simulink model "reconfig"  (R2022a)
settings: Solver=VariableStepAuto  StartTime=0.0  StopTime=tsim  RelTol=1e-3
InitFcn:
  | main
values from neighbouring files (symbols this model uses):
  drone_params = get_parameters(3)    [main.m]
  dt = 0.005    [main.m]
  g = 9.81    [main.m]
  gust_duration = 5    [main.m]
  gust_force = [0;0;0]    [main.m]
  gust_start = 8    [main.m]
  omega0 = [[0,0,0]',[0,0,0]',[0,0,0]']    [main.m]
  p0 = [[0,0,2]',[0,0,2]',[0,0,2]']    [main.m]
  q0 = [[1,0,0,0]',[1,0,0,0]',[1,0,0,0]']    [main.m]
  v0 = [[0,0,0]',[0,0,0]',[0,0,0]']    [main.m]
undefined symbols (not defined in the file or in its folder): dThtdPhidPsi2pqr, pqr2dThtdPhidPsi
libraries: vrlib x1
settings Model: Creator=gbattaglia2021  LastModifiedBy=Giacomo Battaglia
settings DebuggingCC: UnconnectedInputMsg=warning  UnconnectedOutputMsg=warning  UnconnectedLineMsg=warning
settings RTWCC: DLArmComputeVersion=19.05

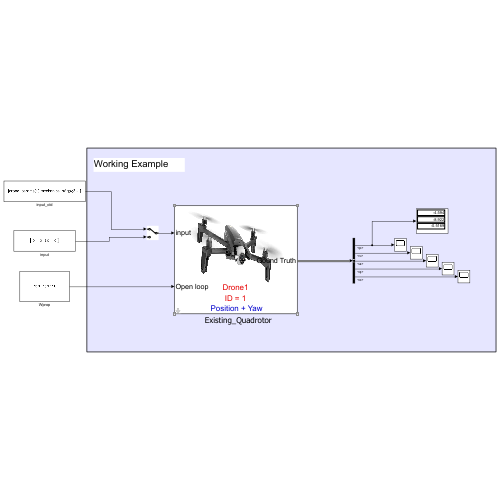
[thumbnail: Simulink's stored preview of the top-level diagram]
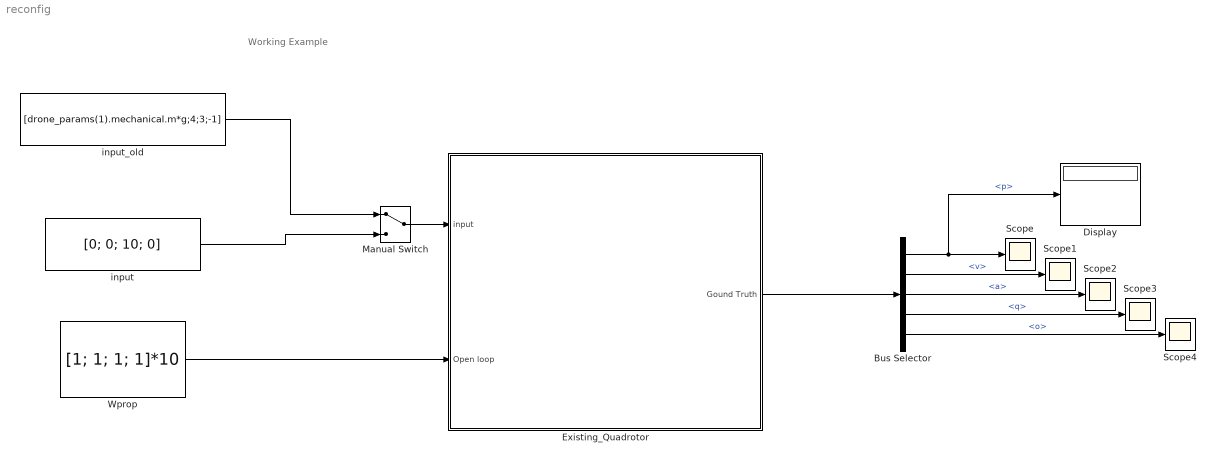
== system reconfig ==
  note: Working Example
  "  Existing_Quadrotor" : Subsystem  mask{control_type_param=1: Position + Yaw, DroneID=1, DroneName=Drone1, idx_offset=0}
      mask prompts: control_type_param "Controller type"; DroneName "Drone Name"; idx_offset "Index Offset"
      mask TypeOptions control_type_param: 1: Position + Yaw | 2: Body Velocity + Yawrate | 3: Body Acceleration + Yawrate | 4: Thrust + Attitude | 5: Thrust + Body Rate | 6: Body Wrench
      mask TypeOptions DroneID: 1 | 2 | 3 | 4 | 5 | 6 | 7 | 8 | 9
      mask Callback DroneID:
      | ID = get_param(gcb,'DroneID');
      | offset = get_param(gcb,'idx_offset');
      | if ischar(ID)
      |   ID = str2num(ID);
      | end
      | if ischar(offset)
      |   offset = str2num(offset);
      | end
      | nameID = ID + offset;
      | set_param(gcb,'DroneName',["Drone"+num2str(nameID)]);
      mask Callback DroneName: set_param([gcb,'/To Workspace'],'VariableName',[get_param(gcb,'DroneName')]);
      mask Callback idx_offset:
      | ID = get_param(gcb,'DroneID');
      | offset = get_param(gcb,'idx_offset');
      | if ischar(ID)
      |   ID = str2num(ID);
      | end
      | if ischar(offset)
      |   offset = str2num(offset);
      | end
      | nameID = ID + offset;
      | set_param(gcb,'DroneName',["Drone"+num2str(nameID)]);
      mask DialogControl Control4 Prompt: click to choose controller
      mask Display:
      | image('format/drone_image.png'); % Use "Edit Image" on toolstrip to change.
      | Name = get_param(gcb,'DroneName');
      | ID = get_param(gcb,'DroneID');
      | C_mode = get_param(gcb,'control_type_param');
      | C_mode(1:2) = [];
      | color('red')
      | ID = "ID = "+ID;
      | color('red')
      | text(0.5, 0.25, Name, 'horizontalAlignment', 'center')
      | color('red')
      | text(0.5, 0.15, ID, 'horizontalAlignment', 'center')
      | color('blue');
      | text(0.5, 0.05, C_mode, 'horizontalAlignment', 'center')
  Bus Selector : BusSelector  OutputSignals=p,v,a,q,o
  Display : Display
  Manual Switch : ManualSwitch
  Scope{,1..4} (5 alike) : Scope
  Wprop : Constant  Value=[1; 1; 1; 1]*10
  input : Constant  Value=[0; 0; 10; 0]
  input_old : Constant  Value=[drone_params(1).mechanical.m*g;4;3;-1]
  wires:
  Bus Selector/1 -> Display/1, Scope/1  "<p>"
  Bus Selector/4 -> Scope3/1  "<q>"
  Bus Selector/5 -> Scope4/1  "<o>"
  Bus Selector/2 -> Scope1/1  "<v>"
  "  Existing_Quadrotor"/1(Gound Truth) -> Bus Selector/1
  Bus Selector/3 -> Scope2/1  "<a>"
  Wprop/1 -> "  Existing_Quadrotor"/2(Open loop)
  Manual Switch/1 -> "  Existing_Quadrotor"/1(input)
  input_old/1 -> Manual Switch/1
  input/1 -> Manual Switch/2

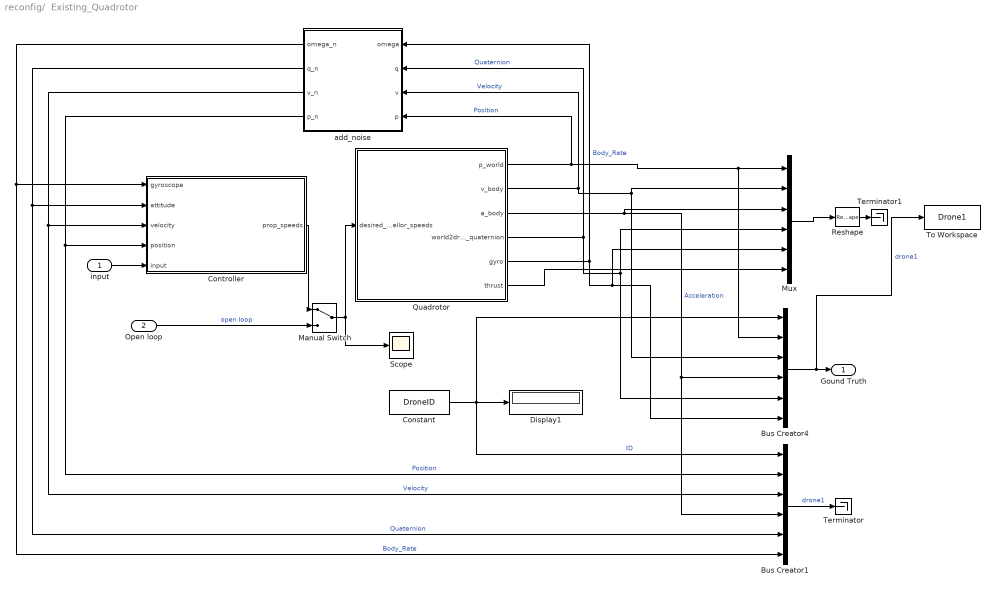
== system reconfig/  Existing_Quadrotor ==
  input : Inport
  Open loop : Inport  Port=2
  Bus Creator1 : BusCreator  Inputs=6  OutDataTypeStr=Bus: DroneStateBus
      settings: InheritFromInputs=off
  Bus Creator4 : BusCreator  Inputs=6  OutDataTypeStr=Bus: DroneStateBus
      settings: InheritFromInputs=off
  Constant : Constant  Value=DroneID
  Controller : Subsystem
  Display1 : Display
  Manual Switch : ManualSwitch
  Mux : Mux  Inputs=6
  Quadrotor : Subsystem
      mask Display: image('droneHardware.jpeg'); % Use "Edit Image" on toolstrip to change.
  Reshape : Reshape
  Scope : Scope
  Terminator : Terminator
  Terminator1 : Terminator
  To Workspace : ToWorkspace  VariableName=Drone1  SaveFormat=Timeseries  SampleTime=-1
  add_noise : MATLAB Function  TreatAsAtomicUnit=on
  Gound Truth : Outport
  wires:
  Quadrotor/5(gyro) -> add_noise/1(omega), Bus Creator4/6, Mux/5  "Body_Rate"
  Quadrotor/1(p_world) -> add_noise/4(p), Bus Creator4/2, Mux/1  "Position"
  Quadrotor/4(world2drone_quaternion) -> add_noise/2(q), Bus Creator4/5, Mux/4  "Quaternion"
  Mux/1 -> Reshape/1
  Quadrotor/2(v_body) -> add_noise/3(v), Bus Creator4/3, Mux/2  "Velocity"
  Quadrotor/6(thrust) -> Mux/6
  input/1 -> Controller/5(input)
  Bus Creator4/1 -> To Workspace/1, Gound Truth/1  "drone1"
  add_noise/2(q_n) -> Bus Creator1/5, Controller/2(attitude)  "Quaternion"
  Quadrotor/3(a_body) -> Mux/3, Bus Creator4/4, Bus Creator1/4  "Acceleration"
  Bus Creator1/1 -> Terminator/1  "drone1"
  add_noise/4(p_n) -> Bus Creator1/2, Controller/4(position)  "Position"
  add_noise/3(v_n) -> Controller/3(velocity), Bus Creator1/3  "Velocity"
  Constant/1 -> Bus Creator4/1, Display1/1, Bus Creator1/1  "ID"
  add_noise/1(omega_n) -> Controller/1(gyroscope), Bus Creator1/6  "Body_Rate"
  Reshape/1 -> Terminator1/1
  Manual Switch/1 -> Scope/1, Quadrotor/1(desired_propellor_speeds)
  Controller/1(prop_speeds) -> Manual Switch/1
  Open loop/1 -> Manual Switch/2  "open loop"

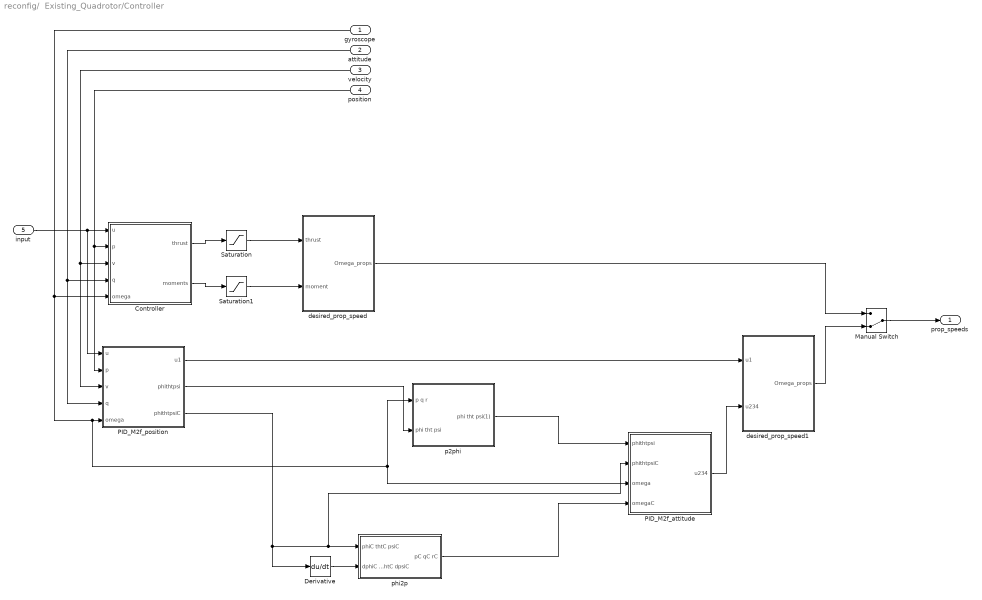
== system reconfig/  Existing_Quadrotor/Controller ==
  gyroscope : Inport
  attitude : Inport  Port=2
  velocity : Inport  Port=3
  position : Inport  Port=4
  input : Inport  Port=5
  Controller : MATLAB Function  TreatAsAtomicUnit=on
  Derivative : Derivative
  Manual Switch : ManualSwitch  CurrentSetting=0
  PID_M2f_attitude : MATLAB Function  TreatAsAtomicUnit=on
  PID_M2f_position : MATLAB Function  TreatAsAtomicUnit=on
  Saturation : Saturate  UpperLimit=16  LowerLimit=3
  Saturation1 : Saturate  UpperLimit=0.1  LowerLimit=-0.1
  desired_prop_speed : MATLAB Function  TreatAsAtomicUnit=on
  desired_prop_speed1 : MATLAB Function  TreatAsAtomicUnit=on
  p2phi : Subsystem
  phi2p : Subsystem
  prop_speeds : Outport
  wires:
  Controller/2(moments) -> Saturation1/1
  Saturation/1 -> desired_prop_speed/1(thrust)
  velocity/1 -> PID_M2f_position/3(v), Controller/3(v)
  Saturation1/1 -> desired_prop_speed/2(moment)
  Controller/1(thrust) -> Saturation/1
  position/1 -> PID_M2f_position/2(p), Controller/2(p)
  input/1 -> Controller/1(u), PID_M2f_position/1(u)
  attitude/1 -> PID_M2f_position/4(q), Controller/4(q)
  gyroscope/1 -> p2phi/1(p q r), PID_M2f_attitude/3(omega), PID_M2f_position/5(omega), Controller/5(omega)
  Manual Switch/1 -> prop_speeds/1
  desired_prop_speed/1(Omega_props) -> Manual Switch/1
  desired_prop_speed1/1(Omega_props) -> Manual Switch/2
  PID_M2f_position/1(u1) -> desired_prop_speed1/1(u1)
  PID_M2f_attitude/1(u234) -> desired_prop_speed1/2(u234)
  PID_M2f_position/2(phithtpsi) -> p2phi/2(phi tht psi)
  p2phi/1(phi tht psi(1)) -> PID_M2f_attitude/1(phithtpsi)
  phi2p/1(pC qC rC) -> PID_M2f_attitude/4(omegaC)
  PID_M2f_position/3(phithtpsiC) -> Derivative/1, PID_M2f_attitude/2(phithtpsiC), phi2p/1(phiC thtC psiC)
  Derivative/1 -> phi2p/2(dphiC dthtC dpsiC)

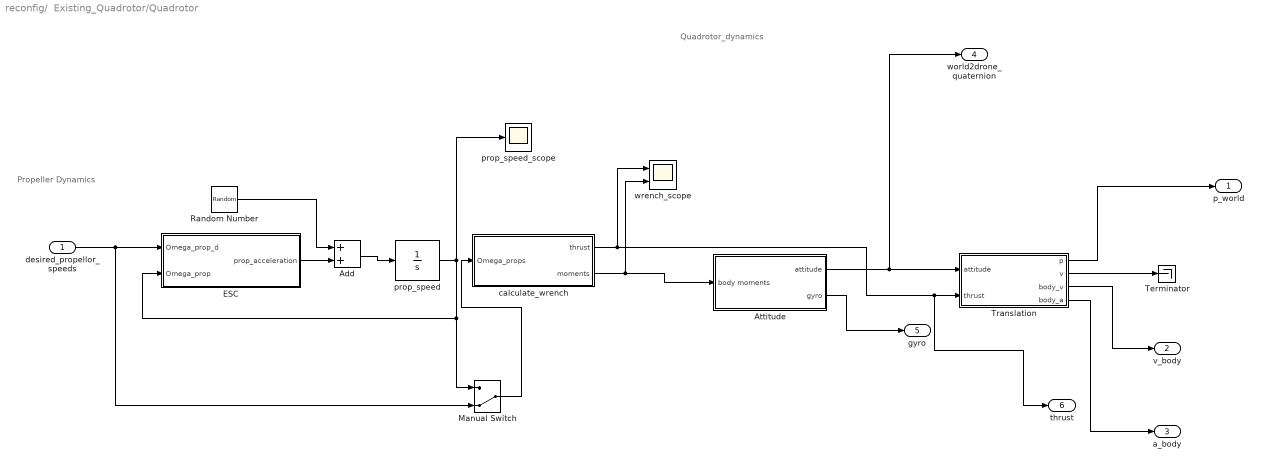
== system reconfig/  Existing_Quadrotor/Quadrotor ==
  note: Quadrotor_dynamics
  note: Propeller Dynamics
  desired_propellor_speeds : Inport
  Add : Sum
  Attitude : Subsystem
  ESC : MATLAB Function  TreatAsAtomicUnit=on
  Manual Switch : ManualSwitch  CurrentSetting=0
  Random Number : RandomNumber  Mean=[0;0;0;0]  Variance=[5000;5000;5000;5000]  Seed=[1;2;3;4]  SampleTime=dt
  Terminator : Terminator
  Translation : Subsystem
  calculate_wrench : MATLAB Function  TreatAsAtomicUnit=on
  prop_speed : Integrator  InitialCondition=drone_params(DroneID).motors.omega0  LimitOutput=on  UpperSaturationLimit=drone_params(DroneID).motors.omega_max  LowerSaturationLimit=drone_params(DroneID).motors.omega_min
  prop_speed_scope : Scope
  wrench_scope : Scope  NumInputPorts=2
  p_world : Outport
  v_body : Outport  Port=2
  a_body : Outport  Port=3
  world2drone_quaternion : Outport  Port=4
  gyro : Outport  Port=5
  thrust : Outport  Port=6
  wires:
  calculate_wrench/1(thrust) -> wrench_scope/1, thrust/1, Translation/2(thrust)
  Add/1 -> prop_speed/1
  desired_propellor_speeds/1 -> Manual Switch/2, ESC/1(Omega_prop_d)
  prop_speed/1 -> Manual Switch/1, ESC/2(Omega_prop), prop_speed_scope/1
  calculate_wrench/2(moments) -> wrench_scope/2, Attitude/1(body moments)
  Attitude/1(attitude) -> world2drone_quaternion/1, Translation/1(attitude)
  Attitude/2(gyro) -> gyro/1
  Translation/3(body_v) -> v_body/1
  Translation/4(body_a) -> a_body/1
  Translation/1(p) -> p_world/1
  Random Number/1 -> Add/1
  ESC/1(prop_acceleration) -> Add/2
  Manual Switch/1 -> calculate_wrench/1(Omega_props)
  Translation/2(v) -> Terminator/1

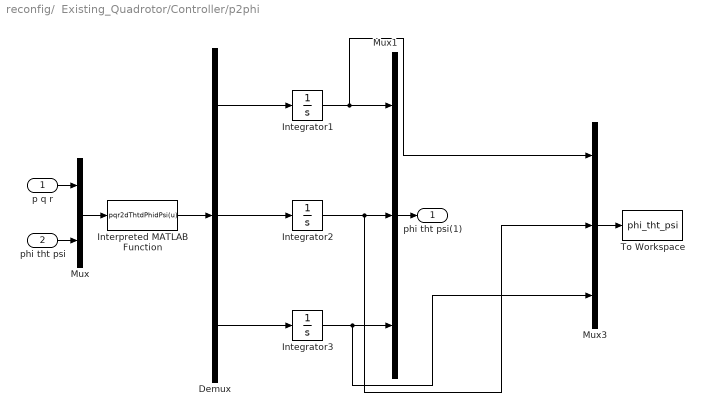
== system reconfig/  Existing_Quadrotor/Controller/p2phi ==
  p q r : Inport
  phi tht psi : Inport  Port=2
  Demux : Demux  Outputs=3
  Integrator1 : Integrator
  Integrator2 : Integrator
  Integrator3 : Integrator
  Interpreted MATLAB Function : MATLABFcn  MATLABFcn=pqr2dThtdPhidPsi(u)  OutputDimensions=3
  Mux : Mux  Inputs=2
  Mux1 : Mux  Inputs=3
  Mux3 : Mux  Inputs=3
  To Workspace : ToWorkspace  VariableName=phi_tht_psi  SampleTime=-1
  phi tht psi(1) : Outport
  wires:
  Integrator3/1 -> Mux3/3, Mux1/3
  Mux1/1 -> phi tht psi(1)/1
  Interpreted MATLAB Function/1 -> Demux/1
  Demux/3 -> Integrator3/1
  Demux/1 -> Integrator1/1
  Mux/1 -> Interpreted MATLAB Function/1
  Demux/2 -> Integrator2/1
  Integrator1/1 -> Mux3/1, Mux1/1
  phi tht psi/1 -> Mux/2
  p q r/1 -> Mux/1
  Integrator2/1 -> Mux3/2, Mux1/2
  Mux3/1 -> To Workspace/1

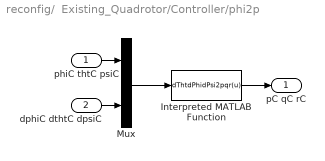
== system reconfig/  Existing_Quadrotor/Controller/phi2p ==
  phiC thtC psiC : Inport
  dphiC dthtC dpsiC : Inport  Port=2
  Interpreted MATLAB Function : MATLABFcn  MATLABFcn=dThtdPhidPsi2pqr(u)  OutputDimensions=3
  Mux : Mux  Inputs=2
  pC qC rC : Outport
  wires:
  Mux/1 -> Interpreted MATLAB Function/1
  phiC thtC psiC/1 -> Mux/1
  Interpreted MATLAB Function/1 -> pC qC rC/1
  dphiC dthtC dpsiC/1 -> Mux/2

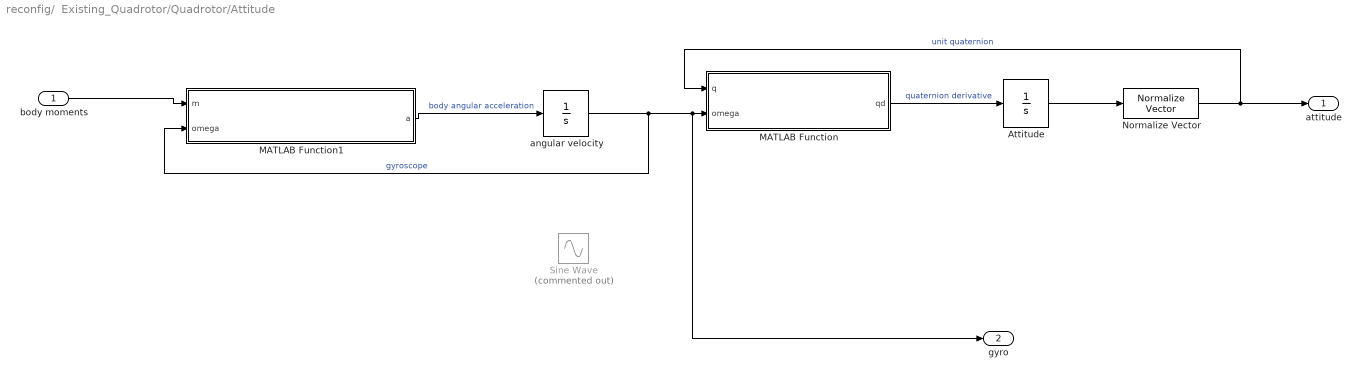
== system reconfig/  Existing_Quadrotor/Quadrotor/Attitude ==
  body moments : Inport
  Attitude : Integrator  InitialCondition=q0(:,DroneID)
  MATLAB Function : MATLAB Function  TreatAsAtomicUnit=on
  MATLAB Function1 : MATLAB Function  TreatAsAtomicUnit=on
  Normalize Vector : vrlib/Utilities/Normalize Vector  maxzero=0
  Sine Wave : Sin  Commented=on  Amplitude=[0.5;0.5;0.5]  Frequency=[1;0.3;0.6]  SampleTime=0
  angular velocity : Integrator  InitialCondition=omega0(:,DroneID)
  attitude : Outport
  gyro : Outport  Port=2
  wires:
  Attitude/1 -> Normalize Vector/1
  MATLAB Function/1(qd) -> Attitude/1  "quaternion derivative"
  body moments/1 -> MATLAB Function1/1(m)
  MATLAB Function1/1(a) -> angular velocity/1  "body angular acceleration"
  angular velocity/1 -> gyro/1, MATLAB Function/2(omega), MATLAB Function1/2(omega)  "gyroscope"
  Normalize Vector/1 -> MATLAB Function/1(q), attitude/1  "unit quaternion"

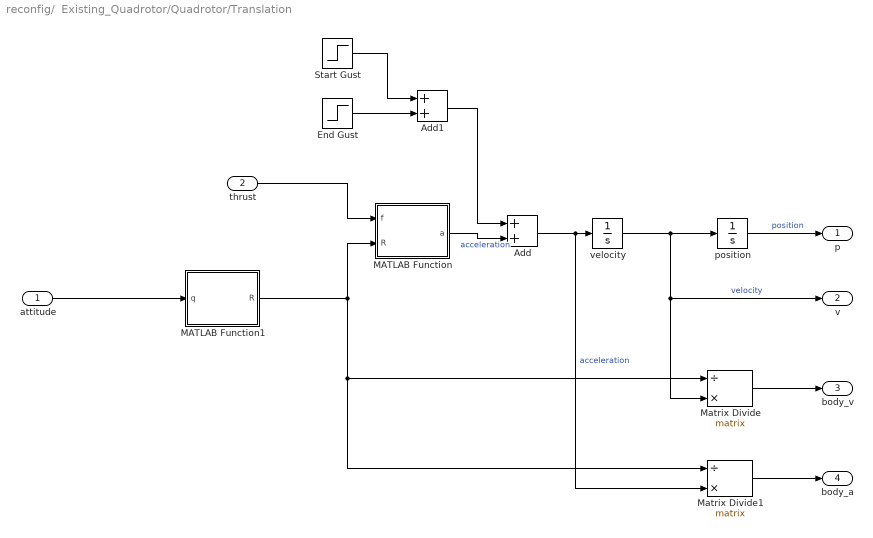
== system reconfig/  Existing_Quadrotor/Quadrotor/Translation ==
  attitude : Inport
  thrust : Inport  Port=2
  Add : Sum
  Add1 : Sum
  End Gust : Step  Time=gust_start + gust_duration  Before=[0;0;0]  After=-1*gust_force/drone_params(DroneID).mechanical.m  SampleTime=0
  MATLAB Function : MATLAB Function  TreatAsAtomicUnit=on
  MATLAB Function1 : MATLAB Function  TreatAsAtomicUnit=on
  Matrix Divide : Product  Inputs=/*  Multiplication=Matrix(*)
  Matrix Divide1 : Product  Inputs=/*  Multiplication=Matrix(*)
  Start Gust : Step  Time=gust_start  Before=[0;0;0]  After=gust_force/drone_params(DroneID).mechanical.m  SampleTime=0
  position : Integrator  InitialCondition=p0(:,DroneID)
  velocity : Integrator  InitialCondition=v0(:,DroneID)
  p : Outport
  v : Outport  Port=2
  body_v : Outport  Port=3
  body_a : Outport  Port=4
  wires:
  velocity/1 -> Matrix Divide/2, v/1, position/1  "velocity"
  position/1 -> p/1  "position"
  Add/1 -> Matrix Divide1/2, velocity/1  "acceleration"
  attitude/1 -> MATLAB Function1/1(q)
  thrust/1 -> MATLAB Function/1(f)
  MATLAB Function1/1(R) -> Matrix Divide1/1, Matrix Divide/1, MATLAB Function/2(R)
  Matrix Divide/1 -> body_v/1
  Matrix Divide1/1 -> body_a/1
  MATLAB Function/1(a) -> Add/2  "acceleration"
  Add1/1 -> Add/1
  End Gust/1 -> Add1/2
  Start Gust/1 -> Add1/1

== matlab function reconfig/  Existing_Quadrotor/Quadrotor/Attitude/MATLAB Function1 ==
  data: m input; a output; omega input; drone_params parameter; DroneID parameter
function a = moments2angularacceleration(m, omega, drone_params, DroneID)

I = drone_params(DroneID).mechanical.I;
a = inv(I)*m  - inv(I) * cross(omega,I*omega);

== matlab function reconfig/  Existing_Quadrotor/Quadrotor/ESC ==
  data: Omega_prop_d input; prop_acceleration output; Omega_prop input; DroneID parameter; drone_params parameter
function prop_acceleration  =  ESC_ctrl(Omega_prop_d, Omega_prop, DroneID, drone_params)

prop_acceleration = (Omega_prop_d - Omega_prop)*drone_params(DroneID).motors.gain;

== matlab function reconfig/  Existing_Quadrotor/Quadrotor/Translation/MATLAB Function ==
  data: f input; a output; R input; g parameter; drone_params parameter; DroneID parameter
function a = fcn(f, R, g, drone_params, DroneID)
m = drone_params(DroneID).mechanical.m;
a = R*[0;0;f]/m - [0;0;g];

== matlab function reconfig/  Existing_Quadrotor/Quadrotor/Translation/MATLAB Function1 ==
  data: q input; R output
function R = quat2rotm(q)
  R = eye(3);
  coder.extrinsic('quat2rotm.m');
  R = quat2rotm(q);
end

== matlab function reconfig/  Existing_Quadrotor/Quadrotor/calculate_wrench ==
  data: Omega_props input; thrust output; moments output; drone_params parameter; DroneID parameter
function [thrust, moments] =  invAllocation(Omega_props, drone_params, DroneID)

wrench = drone_params(DroneID).control.allocation_matrix*Omega_props.^2;

thrust = wrench(1);
moments = wrench(2:4);

== matlab function reconfig/  Existing_Quadrotor/add_noise ==
  settings: updateMethod=DISCRETE
  data: omega input; omega_n output size=3; q input; v input; p input; q_n output size=4; v_n output size=3; p_n output size=3; drone_params parameter; DroneID parameter
function [omega_n, q_n, v_n, p_n]= add_noise(omega,q,v,p, drone_params, DroneID)

omega_n = omega + drone_params(DroneID).sensor.gyroscope_noise*(rand(3,1)-0.5);

q_n = q + drone_params(DroneID).sensor.attitude_noise*(rand(4,1)-0.5);
q_n = q_n/norm(q_n);

v_n = v + drone_params(DroneID).sensor.velocity_noise*(rand(3,1)-0.5);

p_n = p + drone_params(DroneID).sensor.position_noise*(rand(3,1)-0.5);

end

== matlab function reconfig/  Existing_Quadrotor/Controller/PID_M2f_position ==
  data: u input; p input size=3; v input size=3; q input size=4; omega input size=3; u1 output size=1; control_type_param parameter; drone_params parameter; DroneID parameter; g parameter; phithtpsi output; phithtpsiC output
function [u1, phithtpsi, phithtpsiC]   = controller(u, p, v, q, omega, control_type_param, drone_params, DroneID, g)

    R = eye(3);
    coder.extrinsic('quat2rotm.m');
    R = quat2rotm(q);
    angs = rotm2eul(R);
    phi = angs(3);
    tht = angs(2);
    psi = angs(1);

    phithtpsi = [phi; tht; psi];
    
    Kdx = 10; Kpx = 100;
    Kdy = 10; Kpy = 100;
    Kdz = 10; Kpz = 100;
%     Kpphi = 100; Kdphi = 0;
%     Kptht = 100; Kdtht = 0;
%     Kppsi = 100; Kdpsi = 0;
    
    ddxdes = 0;
    ddydes = 0;
    ddzdes = 0;
    dxdes = 0;
    dydes = 0;
    dzdes = 0;
    xdes = u(1);
    ydes = u(2);
    zdes = u(3);
    psides = u(4);
    
    ddxc = ddxdes + Kdx*(dxdes - v(1)) + Kpx*(xdes - p(1));
    ddyc = ddydes + Kdy*(dydes - v(2)) + Kpy*(ydes - p(2));
    ddzc = ddzdes + Kdz*(dzdes - v(3)) + Kpz*(zdes - p(3));
    
%     ddxyzc = [ddxc; ddyc; ddzc];

    phic = 1/g*(ddxc*sin(psides) - ddyc*cos(psides));
    thtc = 1/g*(ddxc*cos(psides) + ddyc*sin(psides));
    psic = psides;

    phithtpsiC = [phic; thtc; psic];

    u1 = drone_params(DroneID).mechanical.m*(g+ddzc);

end

== matlab function reconfig/  Existing_Quadrotor/Controller/desired_prop_speed1 ==
  data: u1 input; Omega_props output; u234 input; drone_params parameter; DroneID parameter
function Omega_props  =  Allocation(u1, u234, drone_params, DroneID)

%  Omega_props = sqrt(inv(alloc_mat) * [thrust;moment]);
%  Omega_props = real(sqrt(complex(inv(drone_params(DroneID).control.allocation_matrix) * [thrust;moment])));

kt = drone_params(DroneID).motors.kt_prop;
kd = drone_params(DroneID).motors.kd_prop;

px = drone_params(DroneID).motors.px;
py = drone_params(DroneID).motors.py;
pz = drone_params(DroneID).motors.pz;

l = drone_params(DroneID).mechanical.l;

P = ...
    [kt         0           kt         0;
     -kt/2      px*kt/l     kt/2       -px*kt/l;
     -kt/2      -py*kt/l    kt/2       py*kt/l;
     -kd        -pz     -kd     -pz];

P = [P(:,2) P(:,4) P(:,1) P(:,3)];

W2 = P \ [u1; u234];
Omega_props = real(sqrt(complex(W2)));

== matlab function reconfig/  Existing_Quadrotor/Controller/PID_M2f_attitude ==
  data: phithtpsi input size=3; phithtpsiC input; omega input size=3; omegaC input size=3; control_type_param parameter; drone_params parameter; DroneID parameter; g parameter; u234 output
function u234   = controller(phithtpsi, phithtpsiC, omega, omegaC, control_type_param, drone_params, DroneID, g)

%     R = eye(3);
%     coder.extrinsic('quat2rotm.m');
%     R = quat2rotm(q);
%     angs = rotm2eul(R);
    phi = phithtpsi(1);
    tht = phithtpsi(2);
    psi = phithtpsi(3);
    
    phic = phithtpsiC(1);
    thtc = phithtpsiC(2);
    psic = phithtpsiC(3);

%     Kdx = 10; Kpx = 10;
%     Kdy = 10; Kpy = 10;
%     Kdz = 10; Kpz = 10;
    Kpphi = 600; Kdphi = 25;
    Kptht = 600; Kdtht = 25;
    Kppsi = 600; Kdpsi = 25;
    
%     ddxdes = 0;
%     ddydes = 0;
%     ddzdes = 0;
%     dxdes = 0;
%     dydes = 0;
%     dzdes = 0;
%     xdes = u(1);
%     ydes = u(2);
%     zdes = u(3);
%     psides = 0;
    
%     ddxc = ddxyzc(1);
%     ddyc = ddxyzc(2);
% 
%     phic = 1/g*(ddxc*sin(psides) - ddyc*cos(psides));
%     thtc = 1/g*(ddxc*cos(psides) + ddyc*sin(psides));
%     psic = psides;

    pc = omegaC(1);
    qc = omegaC(2);
    rc = omegaC(3);

%     u1 = drone_params(DroneID).mechanical.m*(g+ddzc);

    u234 = drone_params(DroneID).mechanical.I*...
        [Kpphi*(phic - phi) + Kdphi*(pc - omega(1));
         Kptht*(thtc - tht) + Kdtht*(qc - omega(2));
         Kppsi*(psic - psi) + Kdpsi*(rc - omega(3));];

end

== matlab function reconfig/  Existing_Quadrotor/Controller/Controller ==
  data: u input; p input size=3; v input size=3; q input size=4; omega input size=3; thrust output size=1; moments output size=3; control_type_param parameter; drone_params parameter; DroneID parameter; g parameter
function [thrust, moments] = controller(u, p, v, q, omega, control_type_param, drone_params, DroneID, g)

    thrust = 1; % set output dim
    moments = [0;0;0]; % set output dim

  coder.extrinsic('droneControl'); % link simulink to matlab function
  
  % do control
  [thrust, moments] = droneControl(u, p, v, q, omega, ...
    control_type_param, drone_params, DroneID, g);


end

== matlab function reconfig/  Existing_Quadrotor/Controller/desired_prop_speed ==
  data: thrust input; Omega_props output; moment input; drone_params parameter; DroneID parameter
function Omega_props  =  Allocation(thrust, moment, drone_params, DroneID)

%  Omega_props = sqrt(inv(alloc_mat) * [thrust;moment]);
 Omega_props = real(sqrt(complex(inv(drone_params(DroneID).control.allocation_matrix) * [thrust;moment])));

== matlab function reconfig/  Existing_Quadrotor/Quadrotor/Attitude/MATLAB Function ==
  data: q input size=4; omega input size=3; qd output size=4
function qd  = quaternion_derivative(q, omega)


qd =  0.5 * multiplyQuaternions([0;omega],q);

end


function q = multiplyQuaternions(qA,qB)
q0 = qA(1);
q1 = qA(2);
q2 = qA(3);
q3 = qA(4);
Q = [q0, -q1, -q2, -q3;
     q1,  q0, -q3,  q2;
     q2,  q3,  q0, -q1;
     q3, -q2,  q1,  q0];
q = Q * qB;
end
